simulink model "pi_2"  (Simulink 6.0)
settings: Solver=ode45  StartTime=0.0  StopTime=20  RelTol=1e-3
undefined symbols (not defined in the file): DiscIntNeverNeededParam
settings Model: LastModifiedBy=star

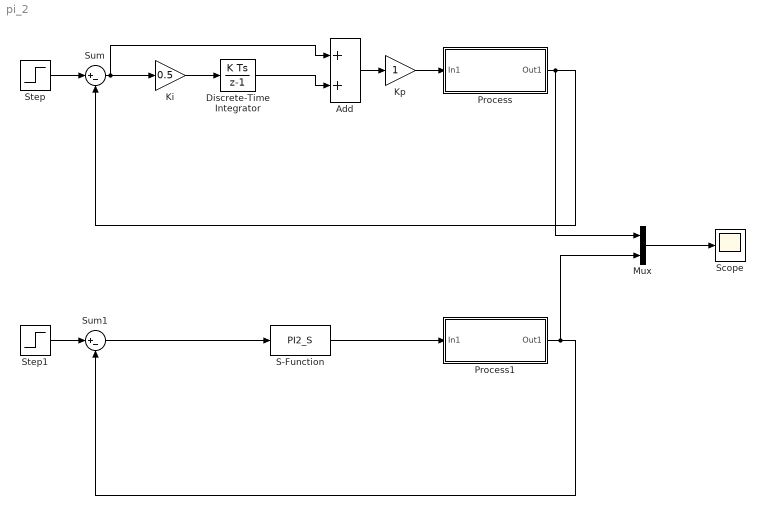
== system pi_2 ==
  Add : Sum  OutScaling=2^-10  SampleTime=0.02
  Discrete-Time Integrator : DiscreteIntegrator  SampleTime=0.02  ICPrevOutput=DiscIntNeverNeededParam  ICPrevScaledInput=DiscIntNeverNeededParam
  Ki : Gain  Gain=0.5  SampleTime=0.02
  Kp : Gain  SampleTime=0.02
  Mux : Mux  Inputs=2
  Process : Subsystem
  Process1 : Subsystem
  S-Function : S-Function  FunctionName=PI2_S  Parameters=0.02, 1, 0.5
  Scope : Scope
  Step : Step  Time=0  SampleTime=0
  Step1 : Step  Time=0  SampleTime=0
  Sum : Sum  Inputs=|+-
  Sum1 : Sum  Inputs=|+-
  wires:
  Sum/1 -> Ki/1, Add/1
  Discrete-Time Integrator/1 -> Add/2
  Ki/1 -> Discrete-Time Integrator/1
  Process/1(Out1) -> Sum/2, Mux/1
  Step/1 -> Sum/1
  Add/1 -> Kp/1
  Kp/1 -> Process/1(In1)
  Process1/1(Out1) -> Sum1/2, Mux/2
  Step1/1 -> Sum1/1
  S-Function/1 -> Process1/1(In1)
  Sum1/1 -> S-Function/1
  Mux/1 -> Scope/1

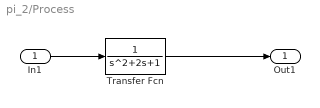
== system pi_2/Process ==
  In1 : Inport  Port=1  LatchInput=off
  Transfer Fcn : TransferFcn
  Out1 : Outport
  wires:
  In1/1 -> Transfer Fcn/1
  Transfer Fcn/1 -> Out1/1

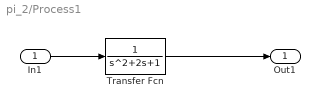
== system pi_2/Process1 ==
  In1 : Inport  Port=1  LatchInput=off
  Transfer Fcn : TransferFcn
  Out1 : Outport
  wires:
  In1/1 -> Transfer Fcn/1
  Transfer Fcn/1 -> Out1/1
